simulink model "Exp_3_13"  (R2024b)
settings: Solver=VariableStepAuto  StartTime=0.0  StopTime=20  RelTol=1e-3
settings Model: Creator=Rj Avro Biswas  LastModifiedBy=Rj Avro Biswas

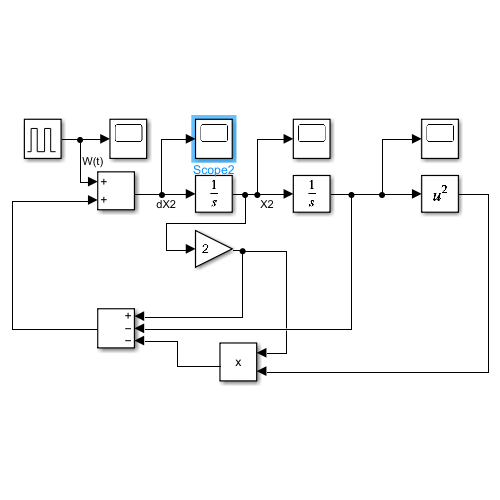
[thumbnail: Simulink's stored preview of the top-level diagram]
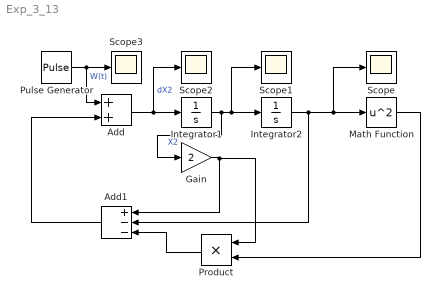
== system Exp_3_13 ==
  Add : Sum
  Add1 : Sum  Inputs=+--
  Gain : Gain  Gain=2
  Integrator1 : Integrator  InitialCondition=2
  Integrator2 : Integrator  InitialCondition=-2
  Math Function : Math  Operator=square
  Product : Product
  Pulse Generator : DiscretePulseGenerator  PulseType=Time based  Amplitude=10  Period=100  PulseWidth=.25
  Scope{,1..3} (4 alike) : Scope
  wires:
  Add/1 -> Scope2/1, Integrator1/1  "dX2"
  Integrator1/1 -> Gain/1, Scope1/1, Integrator2/1  "X2"
  Add1/1 -> Add/2
  Integrator2/1 -> Add1/2, Scope/1, Math Function/1
  Gain/1 -> Product/1, Add1/1
  Product/1 -> Add1/3
  Math Function/1 -> Product/2
  Pulse Generator/1 -> Scope3/1, Add/1  "W(t)"
